simulink model "S12_supra_jza80_rz_stock_v12"  (R2026a)
settings: Solver=FixedStepDiscrete  StopTime=89.98  FixedStep=0.02
undefined symbols (not defined in the file): s12_v12_model_source_step, s12_v12_model_stereo_renderer_step, s12_v12_model_vehicle_cycle_step
settings Model: Creator=Jovi  LastModifiedBy=Jovi

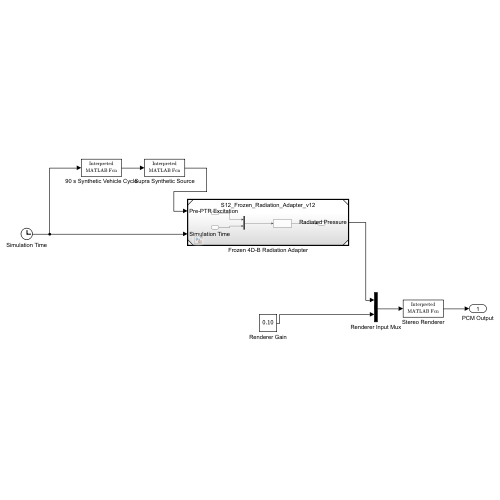
[thumbnail: Simulink's stored preview of the top-level diagram]
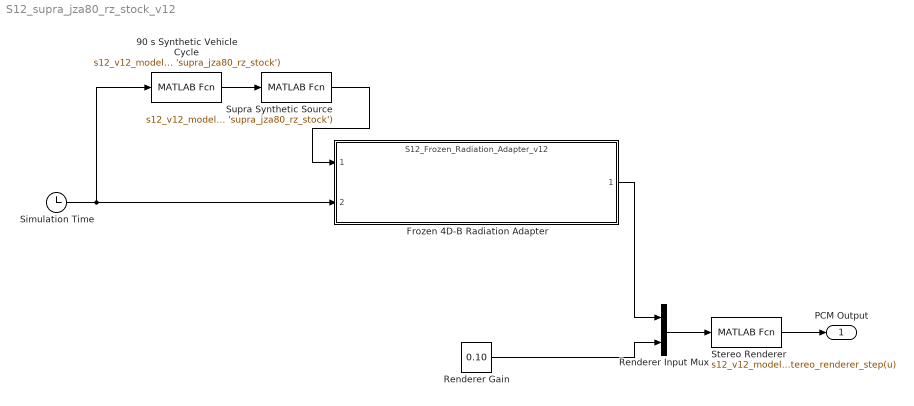
== system S12_supra_jza80_rz_stock_v12 ==
  90 s Synthetic Vehicle Cycle : MATLABFcn  MATLABFcn=s12_v12_model_vehicle_cycle_step(u, 'supra_jza80_rz_stock')  OutputDimensions=[9 1]  Output1D=off
  Frozen 4D-B Radiation Adapter : ModelReference  ModelNameDialog=S12_Frozen_Radiation_Adapter_v12  SimulationMode=Normal  ModelReferenceVersion=1.1
  Renderer Gain : Constant  Value=0.10
  Renderer Input Mux : Mux  Inputs=2
  Simulation Time : Clock
  Stereo Renderer : MATLABFcn  MATLABFcn=s12_v12_model_stereo_renderer_step(u)  OutputDimensions=[960 2]  Output1D=off
  Supra Synthetic Source : MATLABFcn  MATLABFcn=s12_v12_model_source_step(u, 'supra_jza80_rz_stock')  OutputDimensions=[960 1]  Output1D=off
  PCM Output : Outport  PortDimensions=[960 2]
  wires:
  Simulation Time/1 -> Frozen 4D-B Radiation Adapter/2, 90 s Synthetic Vehicle Cycle/1
  90 s Synthetic Vehicle Cycle/1 -> Supra Synthetic Source/1
  Supra Synthetic Source/1 -> Frozen 4D-B Radiation Adapter/1
  Frozen 4D-B Radiation Adapter/1 -> Renderer Input Mux/1
  Renderer Gain/1 -> Renderer Input Mux/2
  Renderer Input Mux/1 -> Stereo Renderer/1
  Stereo Renderer/1 -> PCM Output/1
